simulink model "task6"  (R2022b)
settings: Solver=FixedStepAuto  StartTime=0.0  StopTime=7  RelTol=1e-8
undefined symbols (not defined in the file): k0, k1, k2
settings Model: Creator=anton  LastModifiedBy=anton
settings DataIOCC: ExternalInput=data  LoadExternalInput=on

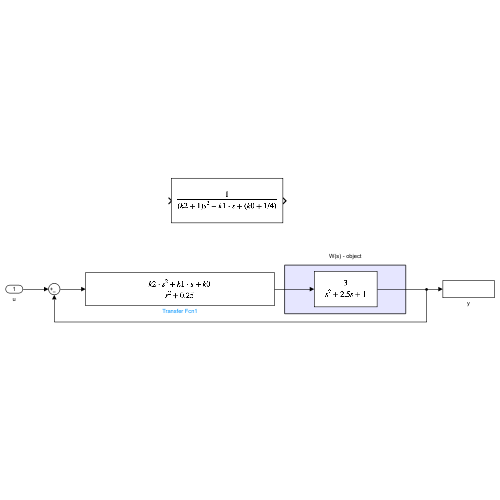
[thumbnail: Simulink's stored preview of the top-level diagram]
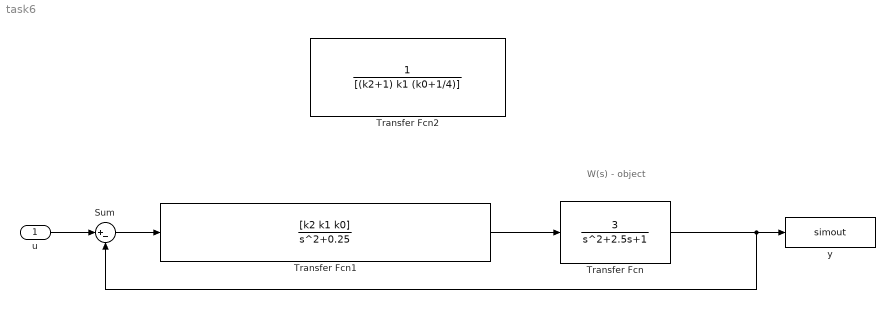
== system task6 ==
  note: W(s) - object
  u : Inport
  Sum : Sum  Inputs=|+-
  Transfer Fcn : TransferFcn  Numerator=[3]  Denominator=[1 2.5 1]
  Transfer Fcn1 : TransferFcn  Numerator=[k2 k1 k0]  Denominator=[1 0 0.25]
  Transfer Fcn2 : TransferFcn  Denominator=[(k2+1) k1 (k0+1/4)]
  y : ToWorkspace  VariableName=simout  SaveFormat=Timeseries  SampleTime=-1
  wires:
  u/1 -> Sum/1
  Transfer Fcn/1 -> Sum/2, y/1
  Transfer Fcn1/1 -> Transfer Fcn/1
  Sum/1 -> Transfer Fcn1/1
